simulink model "mfc"  (R2025a)
settings: Solver=ode45  StartTime=0.0  StopTime=10.0  RelTol=1e-3
settings Model: Creator=Raghuram S  LastModifiedBy=Raghuram S

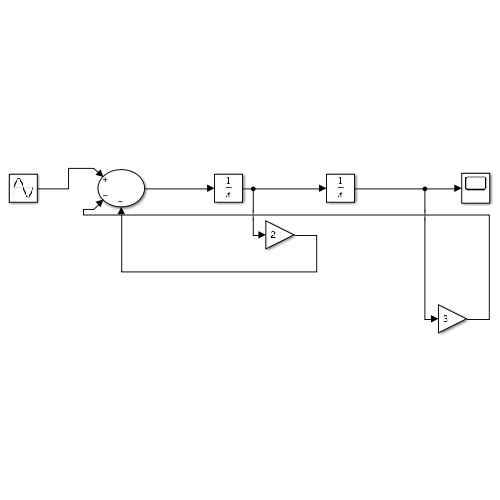
[thumbnail: Simulink's stored preview of the top-level diagram]
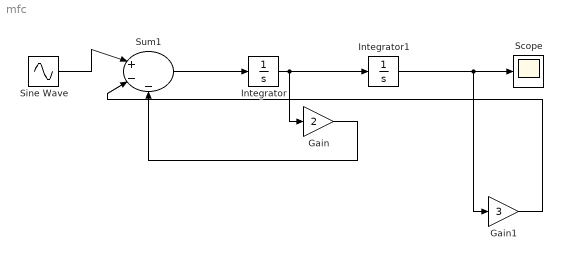
== system mfc ==
  Gain : Gain  Gain=2
  Gain1 : Gain  Gain=3
  Integrator : Integrator
  Integrator1 : Integrator
  Scope : Scope
      settings: ActiveDisplayYMinimum=-0.43990528180878924  ActiveDisplayYMaximum=0.44145811110460548
  Sine Wave : Sin  SampleTime=0
  Sum1 : Sum  Inputs=|+--
  wires:
  Integrator/1 -> Gain/1, Integrator1/1
  Sine Wave/1 -> Sum1/1
  Sum1/1 -> Integrator/1
  Integrator1/1 -> Gain1/1, Scope/1
  Gain/1 -> Sum1/3
  Gain1/1 -> Sum1/2
